simulink model "pneumatiques"  (R2024b)
settings: Solver=FixedStepAuto  StartTime=0.0  StopTime=1  FixedStep=Ts  RelTol=1e-3
settings Model: Creator=marti  LastModifiedBy=marti

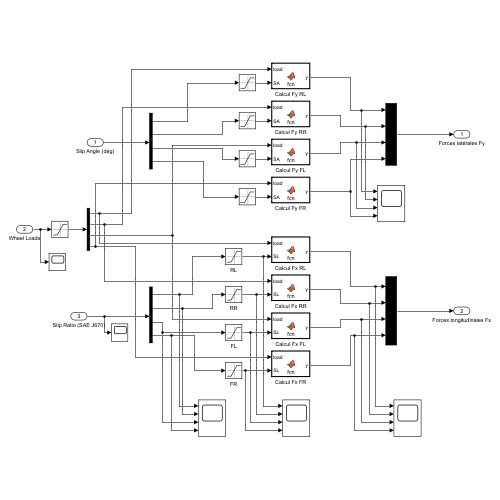
[thumbnail: Simulink's stored preview of the top-level diagram]
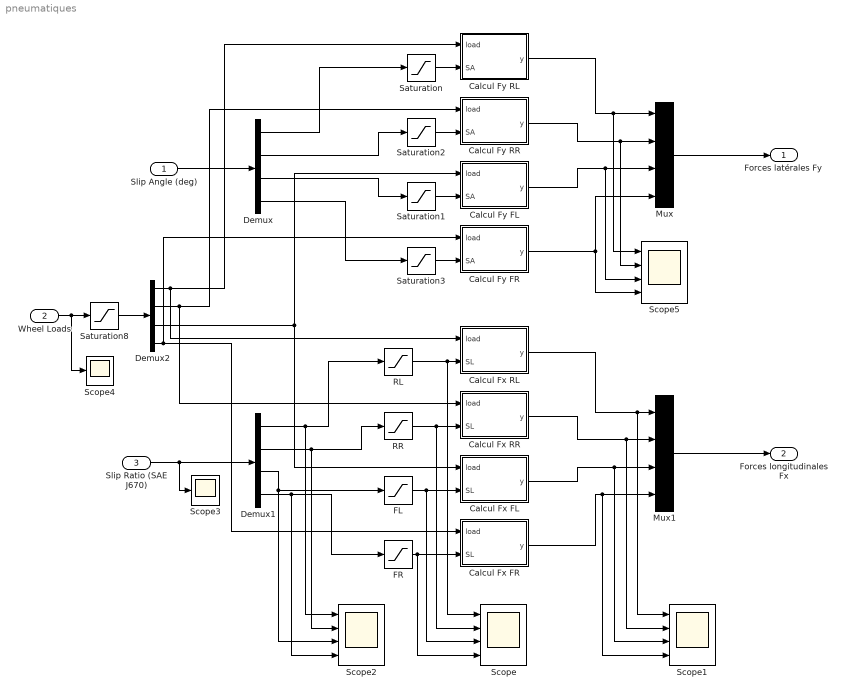
== system pneumatiques ==
  Slip Angle (deg) : Inport
  Wheel Loads : Inport  Port=2
  Slip Ratio (SAE J670) : Inport  Port=3
  Calcul Fx FL : MATLAB Function  TreatAsAtomicUnit=on
  Calcul Fx FR : MATLAB Function  TreatAsAtomicUnit=on
  Calcul Fx RL : MATLAB Function  TreatAsAtomicUnit=on
  Calcul Fx RR : MATLAB Function  TreatAsAtomicUnit=on
  Calcul Fy FL : MATLAB Function  TreatAsAtomicUnit=on
  Calcul Fy FR : MATLAB Function  TreatAsAtomicUnit=on
  Calcul Fy RL : MATLAB Function  TreatAsAtomicUnit=on
  Calcul Fy RR : MATLAB Function  TreatAsAtomicUnit=on
  Demux : Demux
  Demux1 : Demux
  Demux2 : Demux
  FL : Saturate  UpperLimit=0.2  LowerLimit=-0.2
  FR : Saturate  UpperLimit=0.2  LowerLimit=-0.2
  Mux : Mux
  Mux1 : Mux
  RL : Saturate  UpperLimit=0.2  LowerLimit=-0.2
  RR : Saturate  UpperLimit=0.2  LowerLimit=-0.2
  Saturation{,1..3} (4 alike) : Saturate  UpperLimit=8  LowerLimit=-8
  Saturation8 : Saturate  UpperLimit=-300  LowerLimit=-1000
  Scope{,1..2,5} (4 alike) : Scope  NumInputPorts=4
  Scope3 : Scope
  Scope4 : Scope
  Forces latérales Fy : Outport
  Forces longitudinales Fx : Outport  Port=2
  wires:
  Slip Angle (deg)/1 -> Demux/1
  Demux/1 -> Saturation/1
  Demux/2 -> Saturation2/1
  Demux/3 -> Saturation1/1
  Demux/4 -> Saturation3/1
  Slip Ratio (SAE J670)/1 -> Scope3/1, Demux1/1
  Demux1/2 -> Scope2/2, RR/1
  Demux1/4 -> FR/1, Scope2/4
  Demux1/1 -> RL/1, Scope2/1
  Demux1/3 -> FL/1, Scope2/3
  Wheel Loads/1 -> Scope4/1, Saturation8/1
  Demux2/1 -> Calcul Fx RL/1(load), Calcul Fy RL/1(load)
  Demux2/2 -> Calcul Fx RR/1(load), Calcul Fy RR/1(load)
  Demux2/3 -> Calcul Fy FL/1(load), Calcul Fx FL/1(load)
  Demux2/4 -> Calcul Fx FR/1(load), Calcul Fy FR/1(load)
  Calcul Fx RL/1(y) -> Scope1/1, Mux1/1
  Calcul Fx RR/1(y) -> Scope1/2, Mux1/2
  Calcul Fx FL/1(y) -> Scope1/3, Mux1/3
  Calcul Fx FR/1(y) -> Scope1/4, Mux1/4
  Mux1/1 -> Forces longitudinales Fx/1
  Mux/1 -> Forces latérales Fy/1
  Saturation/1 -> Calcul Fy RL/2(SA)
  Saturation1/1 -> Calcul Fy FL/2(SA)
  Saturation2/1 -> Calcul Fy RR/2(SA)
  Saturation3/1 -> Calcul Fy FR/2(SA)
  RL/1 -> Scope/1, Calcul Fx RL/2(SL)
  RR/1 -> Scope/2, Calcul Fx RR/2(SL)
  FL/1 -> Scope/3, Calcul Fx FL/2(SL)
  FR/1 -> Scope/4, Calcul Fx FR/2(SL)
  Saturation8/1 -> Demux2/1
  Calcul Fy RL/1(y) -> Mux/1, Scope5/1
  Calcul Fy FL/1(y) -> Scope5/3, Mux/3
  Calcul Fy FR/1(y) -> Mux/4, Scope5/4
  Calcul Fy RR/1(y) -> Scope5/2, Mux/2

== matlab function pneumatiques/Calcul Fy RL ==
  data: load input; y output; SA input
function y = fcn(load,SA)

y = fonction_pacejka_3D_SA(load,SA);
end

== matlab function pneumatiques/Calcul Fy FR ==
  data: load input; y output; SA input
function y = fcn(load,SA)

y = fonction_pacejka_3D_SA(load,SA);
end

== matlab function pneumatiques/Calcul Fy FL ==
  data: load input; y output; SA input
function y = fcn(load,SA)

y = fonction_pacejka_3D_SA(load,SA);
end

== matlab function pneumatiques/Calcul Fx FL ==
  data: load input; y output; SL input
function y = fcn(load,SL)

y = fonction_pacejka_3D_SL(load,SL);
end

== matlab function pneumatiques/Calcul Fx FR ==
  data: load input; y output; SL input
function y = fcn(load,SL)

y = fonction_pacejka_3D_SL(load,SL);
end

== matlab function pneumatiques/Calcul Fx RL ==
  data: load input; y output; SL input
function y = fcn(load,SL)

y = fonction_pacejka_3D_SL(load,SL);
end

== matlab function pneumatiques/Calcul Fx RR ==
  data: load input; y output; SL input
function y = fcn(load,SL)

y = fonction_pacejka_3D_SL(load,SL);
end

== matlab function pneumatiques/Calcul Fy RR ==
  data: load input; y output; SA input
function y = fcn(load,SA)

y = fonction_pacejka_3D_SA(load,SA);
end
